simulink model "ES90688_p8_1_degrau"  (R2018a)
settings: Solver=FixedStepAuto  StartTime=0.0  StopTime=25  FixedStep=1/100  RelTol=1e-3
libraries: fuzblock x1, simulink x1
settings Model: Creator=Diuary  LastModifiedBy=Diuary

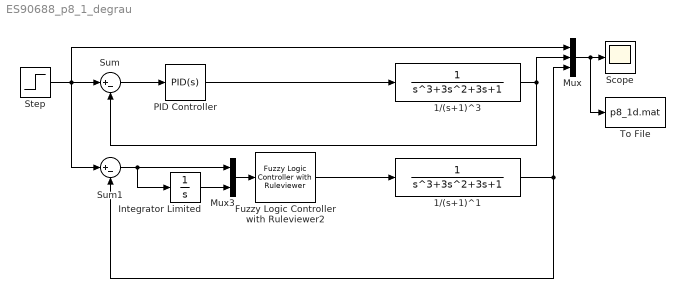
== system ES90688_p8_1_degrau ==
  1/(s+1)^1 : TransferFcn  Denominator=[1 3 3 1]
  1/(s+1)^3 : TransferFcn  Denominator=[1 3 3 1]
  Fuzzy Logic Controller with Ruleviewer2 : fuzblock/Fuzzy Logic  Controller  with Ruleviewer  fismatrix=controle  Ts=0.1
  Integrator Limited : Integrator  LimitOutput=on  UpperSaturationLimit=3  LowerSaturationLimit=-3
  Mux : Mux  Inputs=3
  Mux3 : Mux  Inputs=2
  PID Controller : simulink/Continuous/PID Controller  Controller=PID  TimeDomain=Continuous-time  SampleTime=-1  IntegratorMethod=Forward Euler  FilterMethod=Forward Euler  Form=Parallel  UseFilter=on  ControllerParametersSource=internal  P=2  I=0.5  D=0.05  N=100  InitialConditionSource=internal  InitialConditionForIntegrator=0  InitialConditionForFilter=0  ExternalReset=none  LimitOutput=off  UpperSaturationLimit=inf  LowerSaturationLimit=-inf  LinearizeAsGain=on  AntiWindupMode=none  Kb=1  TrackingMode=off  Kt=1  PParamMin=[]  PParamMax=[]  IParamMin=[]  IParamMax=[]  DParamMin=[]  DParamMax=[]  NParamMin=[]  NParamMax=[]  KbParamMin=[]  KbParamMax=[]  KtParamMin=[]  KtParamMax=[]  POutMin=[]  POutMax=[]  IOutMin=[]  IOutMax=[]  DOutMin=[]  DOutMax=[]  NOutMin=[]  NOutMax=[]  KbOutMin=[]  KbOutMax=[]  KtOutMin=[]  KtOutMax=[]  IntegratorOutMin=[]  IntegratorOutMax=[]  FilterOutMin=[]  FilterOutMax=[]  SumOutMin=[]  SumOutMax=[]  SumI1OutMin=[]  SumI1OutMax=[]  SumI2OutMin=[]  SumI2OutMax=[]  SumI3OutMin=[]  SumI3OutMax=[]  SumDOutMin=[]  SumDOutMax=[]  SaturationOutMin=[]  SaturationOutMax=[]  IntegratorContinuousStateAttributes=''  IntegratorStateMustResolveToSignalObject=off  IntegratorRTWStateStorageClass=Auto  FilterContinuousStateAttributes=''  FilterStateMustResolveToSignalObject=off  FilterRTWStateStorageClass=Auto  DifferentiatorICPrevScaledInput=0  DifferentiatorOutMin=[]  DifferentiatorOutMax=[]  FilterDiffOutCoefMin=[]  FilterDiffOutCoefMax=[]  SumDenOutMin=[]  SumDenOutMax=[]  SumNumOutMin=[]  SumNumOutMax=[]  ReciprocalOutMin=[]  ReciprocalOutMax=[]  DivideOutMin=[]  DivideOutMax=[]  TunerSelectOption=Transfer Function Based (PID Tuner App)
  Scope : Scope
  Step : Step  SampleTime=0
  Sum : Sum  Inputs=|+-
  Sum1 : Sum  Inputs=|+-
  To File : ToFile  Filename=p8_1d.mat  MatrixName=degrau  SaveFormat=Timeseries
  wires:
  PID Controller/1 -> 1/(s+1)^3/1
  Sum/1 -> PID Controller/1
  1/(s+1)^3/1 -> Mux/2, Sum/2
  Mux/1 -> To File/1, Scope/1
  Sum1/1 -> Integrator Limited/1, Mux3/1
  1/(s+1)^1/1 -> Mux/3, Sum1/2
  Step/1 -> Sum1/1, Mux/1, Sum/1
  Mux3/1 -> Fuzzy Logic Controller with Ruleviewer2/1
  Integrator Limited/1 -> Mux3/2
  Fuzzy Logic Controller with Ruleviewer2/1 -> 1/(s+1)^1/1
